simulink model "Check1"  (R2016b)
settings: Solver=VariableStepAuto  StartTime=0.0  StopTime=10.0  RelTol=1e-3
values from neighbouring files (symbols this model uses):
  A1 = 44.1942    [Lab2.m]    (also in step_5.mat)
  A2 = 55.706    [Lab2.m]
  B1 = 3.33541    [Lab2.m]    (also in step_5.mat)
  B2 = 3.16511597    [Lab2.m]
settings Model: Creator=EE103  LastModifiedBy=EE103

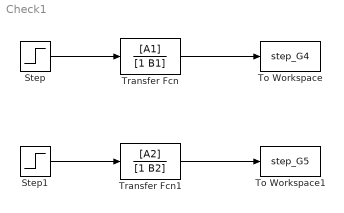
== system Check1 ==
  Step : Step  Time=0  After=4  SampleTime=0.01
  Step1 : Step  Time=0  After=5  SampleTime=0.01
  To Workspace : ToWorkspace  VariableName=step_G4  SaveFormat=Timeseries  SampleTime=-1
  To Workspace1 : ToWorkspace  VariableName=step_G5  SaveFormat=Timeseries  SampleTime=-1
  Transfer Fcn : TransferFcn  Numerator=[A1]  Denominator=[1 B1]
  Transfer Fcn1 : TransferFcn  Numerator=[A2]  Denominator=[1 B2]
  wires:
  Step/1 -> Transfer Fcn/1
  Transfer Fcn/1 -> To Workspace/1
  Step1/1 -> Transfer Fcn1/1
  Transfer Fcn1/1 -> To Workspace1/1
